simulink model "s4"  (Simulink 2.00)
settings: Solver=ode113  StartTime=0.0  StopTime=tstop  MaxStep=1e-3  RelTol=1e-5  AbsTol=1e-5
values from neighbouring files (symbols this model uses):
  Dpsi = [ -2454.6 -2412.6 -2370.5 -2328.5 -2286.4 -2244.4 -2202.3  -2160.3 -2118.2 -2076.1 -2034.1 -1992.0 -1950.0 -1907.9 -1865.9  -1823.8 -1781.8 -1739.7 -1697.7 -1655.6 -1613.6 -1571.5 -1529.5  -1487.4 -1445.3 -1403.3 -1361.2 -1319.2 -1277.1 -1235.1 -1193.0  -1151.0 -1108.9 -1066.9 -1024.8 -982.76 -940.71 -898.65 -856.60  -814.55 -772.49 -730.44 -688.39 -646.43 -604.66 -562.89 -521.30  -479.53 -438.14  ...(+559 chars)    [M1.M]    (also in M4.M)
  NpbyNs = 120/240    (= 0.5)    [M1.M]    (also in M4.M)
  Psi1o = 0    [M1.M]    (also in M4.M)
  Psip2o = 0    [M1.M]    (also in M4.M)
  psisat = [ -170.21 -169.93 -169.65 -169.36 -169.08 -168.80 -168.52  -168.23 -167.95 -167.67 -167.38 -167.10 -166.82 -166.54 -166.25  -165.97 -165.69 -165.40 -165.12 -164.84 -164.56 -164.27 -163.99  -163.71 -163.43 -163.14 -162.86 -162.58 -162.29 -162.01 -161.73  -161.45 -161.16 -160.88 -160.60 -160.32 -160.03 -159.75 -159.47  -159.18 -158.90 -158.62 -158.34 -157.96 -157.39 -156.83 -156.07  -155.51 -154.57  ...(+561 chars)    [M1.M]    (also in M4.M)
  r1 = 0.25    [M1.M]    (also in M4.M)
  Rn = input('Enter ohmic value of neutral to ground resistor Rn > ')    [M4.M]
  rp2 = 0.134    [M1.M]    (also in M4.M)
  wb = 2*pi*Frated    (= 376.991118431)    [M1.M]    (also in M4.M)
  xl1 = 0.056    [M1.M]    (also in M4.M)
  xM = 1/(1/xm + 1/xl1 + 1/xpl2)    (= 0.0279988939489)    [M1.M]    (also in M4.M)
  xm = 708.8    [M1.M]    (also in M4.M)
  xpl2 = 0.056    [M1.M]    (also in M4.M)
settings Model: SaveTime=off  SaveOutput=off  ConsistencyChecking=off

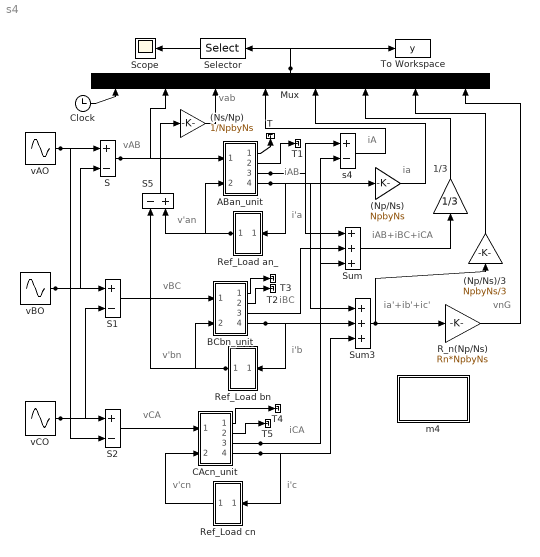
== system s4 ==
  note: vCA
  note: i'a
  note: iAB
  note: iCA
  note: v'bn
  note: vBC
  note: v'cn
  note: i'c
  note: i'b
  note: v'an
  note: iBC
  note: vnG
  note: vab
  note: vAB
  note: iA
  note: ia
  note: iAB+iBC+iCA
  note: ia'+ib'+ic'
  (Np/Ns) : Gain  Gain=NpbyNs
  (Np/Ns)/3 : Gain  Orientation=up  Gain=NpbyNs/3
  (Ns/Np) : Gain  Gain=1/NpbyNs
  1/3 : Gain  Orientation=up  Gain=1/3
  ABan_unit : Subsystem
  BCbn_unit : Subsystem
  CAcn_unit : Subsystem
  Clock : Clock
      settings: DeleteFcn=simclock BlockIsBeingDestroyed  PostSaveFcn=simclock Save
  m4 : Subsystem
      settings: OpenFcn=m4
      mask Type: Masked block of m4.m
      mask Help: Uses m4.m to initialize and plot
      mask Display: disp('Initialize\nand plot')
  Mux : Mux  Orientation=up  Inputs=8
  R_n(Np/Ns) : Gain  Gain=Rn*NpbyNs
  Ref_Load an_ : Subsystem  Orientation=left
  Ref_Load bn : Subsystem  Orientation=left
  Ref_Load cn : Subsystem  Orientation=left
  S : Sum  Inputs=+-
  S1 : Sum  Inputs=+-
  S2 : Sum  Inputs=+-
  s4 : Sum  Inputs=+-
  S5 : Sum  Orientation=up  Inputs=-+
  Scope : Scope
      settings: TickLabels=on  TimeRange=0.1  YMin=-500  YMax=500  SaveToWorkspace=off  SaveName=ScopeData  LimitMaxRows=off
  Selector : Selector  Orientation=left  Elements=[2 3 4 5 6 7]  InputPortWidth=8
  Sum : Sum  Inputs=+++
  Sum3 : Sum  Inputs=+++
  T{,1..5} (6 alike) : Terminator
      T settings: Orientation=up
  To Workspace : ToWorkspace  VariableName=y  SampleTime=0
      settings: Buffer=10000
  vAO : Sin  Amplitude=169.7/sqrt(3)  Frequency=120*pi  Phase=0  SampleTime=-1
  vBO : Sin  Amplitude=169.7/sqrt(3)  Frequency=120*pi  Phase=-2*pi/3  SampleTime=-1
  vCO : Sin  Amplitude=169.7/sqrt(3)  Frequency=120*pi  Phase=-4*pi/3  SampleTime=-1
  wires:
  Clock/1 -> Mux/1
  S1/1 -> BCbn_unit/1(in_1)
  S2/1 -> CAcn_unit/1(in_1)
  Ref_Load cn/1(out_1) -> CAcn_unit/2(in_2)
  BCbn_unit/4(out_i2') -> Ref_Load bn/1(in_1), Sum3/2
  CAcn_unit/4(out_i2') -> Ref_Load cn/1(in_1), Sum3/3
  vBO/1 -> S1/1, S/2
  vCO/1 -> S2/1, S1/2
  vAO/1 -> S/1, S2/2
  ABan_unit/4(out_i2') -> Sum3/1, Ref_Load an_/1(in_1), (Np/Ns)/1
  (Np/Ns)/1 -> Mux/5
  S5/1 -> (Ns/Np)/1
  Ref_Load an_/1(out_1) -> ABan_unit/2(in_2), S5/2
  Ref_Load bn/1(out_1) -> BCbn_unit/2(in_2), S5/1
  s4/1 -> Mux/4
  S/1 -> ABan_unit/1(in_1), Mux/2
  (Ns/Np)/1 -> Mux/3
  ABan_unit/3(out_i1) -> s4/1, Sum/1
  BCbn_unit/3(out_i1) -> Sum/2
  CAcn_unit/3(out_i1) -> s4/2, Sum/3
  R_n(Np/Ns)/1 -> Mux/8
  Sum/1 -> 1/3/1
  1/3/1 -> Mux/6
  (Np/Ns)/3/1 -> Mux/7
  Sum3/1 -> R_n(Np/Ns)/1, (Np/Ns)/3/1
  Selector/1 -> Scope/1
  Mux/1 -> To Workspace/1, Selector/1
  ABan_unit/1(out_psi1) -> T/1
  ABan_unit/2(out_psim) -> T1/1
  BCbn_unit/1(out_psi1) -> T2/1
  BCbn_unit/2(out_psim) -> T3/1
  CAcn_unit/1(out_psi1) -> T4/1
  CAcn_unit/2(out_psim) -> T5/1

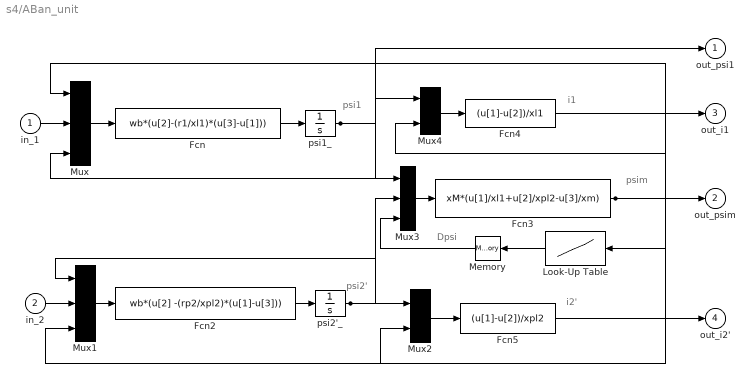
== system s4/ABan_unit ==
  note: i2'
  note: Dpsi
  note: psim
  note: psi2'
  note: psi1
  note: i1
  in_1 : Inport  Port=1  PortWidth=-1  SampleTime=-1
  in_2 : Inport  Port=2  PortWidth=-1  SampleTime=-1
  Fcn : Fcn  Expr=wb*(u[2]-(r1/xl1)*(u[3]-u[1]))
  Fcn2 : Fcn  Expr=wb*(u[2] -(rp2/xpl2)*(u[1]-u[3]))
  Fcn3 : Fcn  Expr=xM*(u[1]/xl1+u[2]/xpl2-u[3]/xm)
  Fcn4 : Fcn  Expr=(u[1]-u[2])/xl1
  Fcn5 : Fcn  Expr=(u[1]-u[2])/xpl2
  Look-Up Table : Lookup  Orientation=left  InputValues=psisat  OutputValues=Dpsi
  Memory : Memory  Orientation=left  X0=0  InheritSampleTime=off
  Mux : Mux  Inputs=3
  Mux1 : Mux  Inputs=3
  Mux2 : Mux  Inputs=2
  Mux3 : Mux  Inputs=3
  Mux4 : Mux  Inputs=2
  psi1_ : Integrator  ExternalReset=none  InitialConditionSource=internal  InitialCondition=Psi1o  LimitOutput=off  UpperSaturationLimit=inf  LowerSaturationLimit=-inf  ShowSaturationPort=off  ShowStatePort=off  AbsoluteTolerance=auto
  psi2'_ : Integrator  ExternalReset=none  InitialConditionSource=internal  InitialCondition=Psip2o  LimitOutput=off  UpperSaturationLimit=inf  LowerSaturationLimit=-inf  ShowSaturationPort=off  ShowStatePort=off  AbsoluteTolerance=auto
  out_psi1 : Outport  Port=1  InitialOutput=0
  out_psim : Outport  Port=2  InitialOutput=0
  out_i1 : Outport  Port=3  InitialOutput=0
  out_i2' : Outport  Port=4  InitialOutput=0
  wires:
  Look-Up Table/1 -> Memory/1
  Memory/1 -> Mux3/3
  Fcn3/1 -> Look-Up Table/1, Mux2/2, Mux/1, Mux1/3, Mux4/2, out_psim/1
  Mux2/1 -> Fcn5/1
  psi2'_/1 -> Mux2/1, Mux3/2, Mux1/1
  Mux1/1 -> Fcn2/1
  psi1_/1 -> Mux/3, Mux4/1, Mux3/1, out_psi1/1
  Mux4/1 -> Fcn4/1
  Mux3/1 -> Fcn3/1
  Fcn2/1 -> psi2'_/1
  Fcn/1 -> psi1_/1
  Mux/1 -> Fcn/1
  Fcn4/1 -> out_i1/1
  in_1/1 -> Mux/2
  in_2/1 -> Mux1/2
  Fcn5/1 -> out_i2'/1

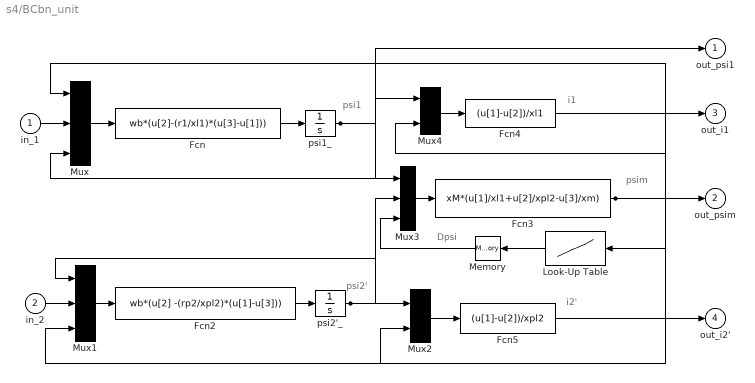
== system s4/BCbn_unit ==
  note: i2'
  note: Dpsi
  note: psim
  note: psi2'
  note: psi1
  note: i1
  in_1 : Inport  Port=1  PortWidth=-1  SampleTime=-1
  in_2 : Inport  Port=2  PortWidth=-1  SampleTime=-1
  Fcn : Fcn  Expr=wb*(u[2]-(r1/xl1)*(u[3]-u[1]))
  Fcn2 : Fcn  Expr=wb*(u[2] -(rp2/xpl2)*(u[1]-u[3]))
  Fcn3 : Fcn  Expr=xM*(u[1]/xl1+u[2]/xpl2-u[3]/xm)
  Fcn4 : Fcn  Expr=(u[1]-u[2])/xl1
  Fcn5 : Fcn  Expr=(u[1]-u[2])/xpl2
  Look-Up Table : Lookup  Orientation=left  InputValues=psisat  OutputValues=Dpsi
  Memory : Memory  Orientation=left  X0=0  InheritSampleTime=off
  Mux : Mux  Inputs=3
  Mux1 : Mux  Inputs=3
  Mux2 : Mux  Inputs=2
  Mux3 : Mux  Inputs=3
  Mux4 : Mux  Inputs=2
  psi1_ : Integrator  ExternalReset=none  InitialConditionSource=internal  InitialCondition=Psi1o  LimitOutput=off  UpperSaturationLimit=inf  LowerSaturationLimit=-inf  ShowSaturationPort=off  ShowStatePort=off  AbsoluteTolerance=auto
  psi2'_ : Integrator  ExternalReset=none  InitialConditionSource=internal  InitialCondition=Psip2o  LimitOutput=off  UpperSaturationLimit=inf  LowerSaturationLimit=-inf  ShowSaturationPort=off  ShowStatePort=off  AbsoluteTolerance=auto
  out_psi1 : Outport  Port=1  InitialOutput=0
  out_psim : Outport  Port=2  InitialOutput=0
  out_i1 : Outport  Port=3  InitialOutput=0
  out_i2' : Outport  Port=4  InitialOutput=0
  wires:
  Look-Up Table/1 -> Memory/1
  Memory/1 -> Mux3/3
  Fcn3/1 -> Look-Up Table/1, Mux2/2, Mux/1, Mux1/3, Mux4/2, out_psim/1
  Mux2/1 -> Fcn5/1
  psi2'_/1 -> Mux2/1, Mux3/2, Mux1/1
  Mux1/1 -> Fcn2/1
  psi1_/1 -> Mux/3, Mux4/1, Mux3/1, out_psi1/1
  Mux4/1 -> Fcn4/1
  Mux3/1 -> Fcn3/1
  Fcn2/1 -> psi2'_/1
  Fcn/1 -> psi1_/1
  Mux/1 -> Fcn/1
  Fcn4/1 -> out_i1/1
  in_1/1 -> Mux/2
  in_2/1 -> Mux1/2
  Fcn5/1 -> out_i2'/1

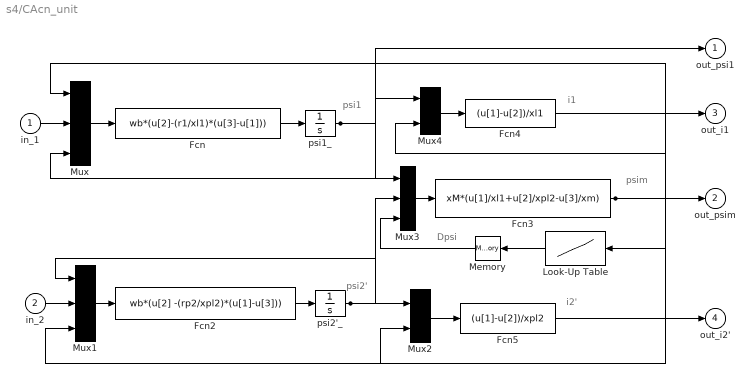
== system s4/CAcn_unit ==
  note: i2'
  note: Dpsi
  note: psim
  note: psi2'
  note: psi1
  note: i1
  in_1 : Inport  Port=1  PortWidth=-1  SampleTime=-1
  in_2 : Inport  Port=2  PortWidth=-1  SampleTime=-1
  Fcn : Fcn  Expr=wb*(u[2]-(r1/xl1)*(u[3]-u[1]))
  Fcn2 : Fcn  Expr=wb*(u[2] -(rp2/xpl2)*(u[1]-u[3]))
  Fcn3 : Fcn  Expr=xM*(u[1]/xl1+u[2]/xpl2-u[3]/xm)
  Fcn4 : Fcn  Expr=(u[1]-u[2])/xl1
  Fcn5 : Fcn  Expr=(u[1]-u[2])/xpl2
  Look-Up Table : Lookup  Orientation=left  InputValues=psisat  OutputValues=Dpsi
  Memory : Memory  Orientation=left  X0=0  InheritSampleTime=off
  Mux : Mux  Inputs=3
  Mux1 : Mux  Inputs=3
  Mux2 : Mux  Inputs=2
  Mux3 : Mux  Inputs=3
  Mux4 : Mux  Inputs=2
  psi1_ : Integrator  ExternalReset=none  InitialConditionSource=internal  InitialCondition=Psi1o  LimitOutput=off  UpperSaturationLimit=inf  LowerSaturationLimit=-inf  ShowSaturationPort=off  ShowStatePort=off  AbsoluteTolerance=auto
  psi2'_ : Integrator  ExternalReset=none  InitialConditionSource=internal  InitialCondition=Psip2o  LimitOutput=off  UpperSaturationLimit=inf  LowerSaturationLimit=-inf  ShowSaturationPort=off  ShowStatePort=off  AbsoluteTolerance=auto
  out_psi1 : Outport  Port=1  InitialOutput=0
  out_psim : Outport  Port=2  InitialOutput=0
  out_i1 : Outport  Port=3  InitialOutput=0
  out_i2' : Outport  Port=4  InitialOutput=0
  wires:
  Look-Up Table/1 -> Memory/1
  Memory/1 -> Mux3/3
  Fcn3/1 -> Look-Up Table/1, Mux2/2, Mux/1, Mux1/3, Mux4/2, out_psim/1
  Mux2/1 -> Fcn5/1
  psi2'_/1 -> Mux2/1, Mux3/2, Mux1/1
  Mux1/1 -> Fcn2/1
  psi1_/1 -> Mux/3, Mux4/1, Mux3/1, out_psi1/1
  Mux4/1 -> Fcn4/1
  Mux3/1 -> Fcn3/1
  Fcn2/1 -> psi2'_/1
  Fcn/1 -> psi1_/1
  Mux/1 -> Fcn/1
  Fcn4/1 -> out_i1/1
  in_1/1 -> Mux/2
  in_2/1 -> Mux1/2
  Fcn5/1 -> out_i2'/1

== system s4/m4 ==
  note: Masked block of m4.m to initilaize s4.m
      | and plot results of simulation

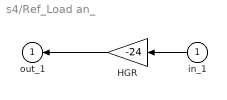
== system s4/Ref_Load an_ ==
  in_1 : Inport  Orientation=left  Port=1  PortWidth=-1  SampleTime=-1
  HGR : Gain  Orientation=left  Gain=-24
  out_1 : Outport  Orientation=left  Port=1  InitialOutput=0
  wires:
  HGR/1 -> out_1/1
  in_1/1 -> HGR/1

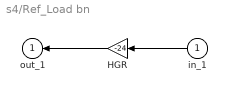
== system s4/Ref_Load bn ==
  in_1 : Inport  Orientation=left  Port=1  PortWidth=-1  SampleTime=-1
  HGR : Gain  Orientation=left  Gain=-24
  out_1 : Outport  Orientation=left  Port=1  InitialOutput=0
  wires:
  HGR/1 -> out_1/1
  in_1/1 -> HGR/1

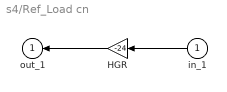
== system s4/Ref_Load cn ==
  in_1 : Inport  Orientation=left  Port=1  PortWidth=-1  SampleTime=-1
  HGR : Gain  Orientation=left  Gain=-24
  out_1 : Outport  Orientation=left  Port=1  InitialOutput=0
  wires:
  HGR/1 -> out_1/1
  in_1/1 -> HGR/1
